simulink model "CO_laborator_04"  (R2023b)
settings: Solver=VariableStepAuto  StartTime=0.0  StopTime=100  RelTol=1e-3
values from neighbouring files (symbols this model uses):
  A = [-0.313, 56.7 0; -0.0139 -0.426 0; 0 56.7 0]    [CO_laborator_04.m]
  B = [0.232; 0.0203; 0]    [CO_laborator_04.m]
  C = [0 0 1]    [CO_laborator_04.m]
  K = lqr(A,B,Q,R)    [CO_laborator_04.m]
  Kx = K(1:3)    [CO_laborator_04.m]
  Kz = K(4)    [CO_laborator_04.m]
  N = length(t)    [CO_laborator_04.m]
settings Model: Creator=ovidiuceoca  LastModifiedBy=ovidiuceoca

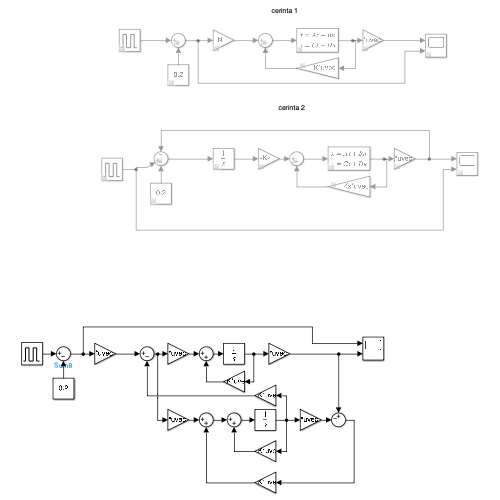
[thumbnail: Simulink's stored preview of the top-level diagram]
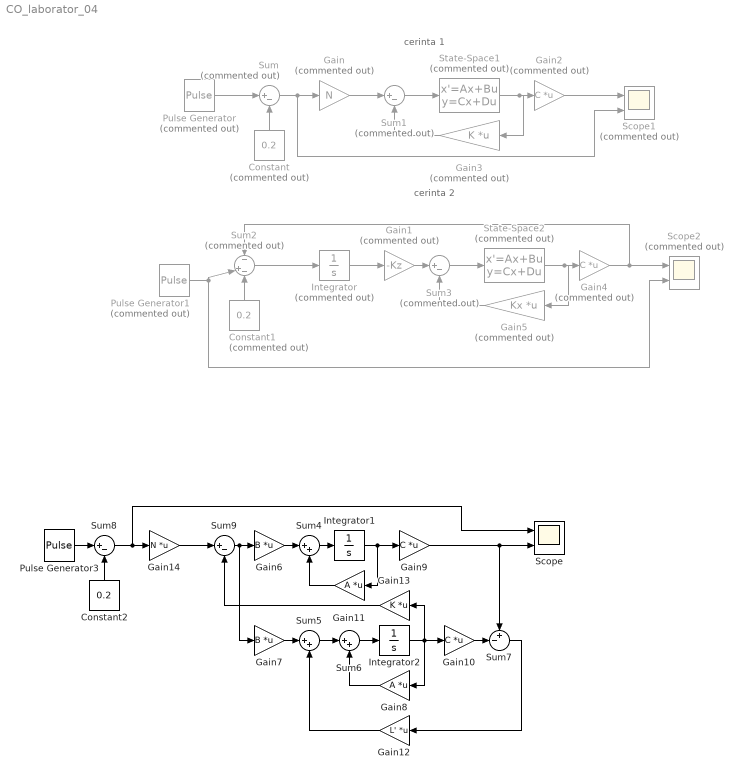
== system CO_laborator_04 ==
  note: cerinta 2
  note: cerinta 1
  Constant : Constant  Commented=on  Value=0.2
  Constant1 : Constant  Commented=on  Value=0.2
  Constant2 : Constant  Value=0.2
  Gain : Gain  Commented=on  Gain=N
  Gain1 : Gain  Commented=on  Gain=-Kz
  Gain10 : Gain  Gain=C  Multiplication=Matrix(K*u) (u vector)
  Gain11 : Gain  Gain=A  Multiplication=Matrix(K*u) (u vector)
  Gain12 : Gain  Gain=L'  Multiplication=Matrix(K*u) (u vector)
  Gain13 : Gain  Gain=K  Multiplication=Matrix(K*u) (u vector)
  Gain14 : Gain  Gain=N  Multiplication=Matrix(K*u) (u vector)
  Gain2 : Gain  Commented=on  Gain=C  Multiplication=Matrix(K*u) (u vector)
  Gain3 : Gain  Commented=on  Gain=K  Multiplication=Matrix(K*u) (u vector)
  Gain4 : Gain  Commented=on  Gain=C  Multiplication=Matrix(K*u) (u vector)
  Gain5 : Gain  Commented=on  Gain=Kx  Multiplication=Matrix(K*u) (u vector)
  Gain6 : Gain  Gain=B  Multiplication=Matrix(K*u) (u vector)
  Gain7 : Gain  Gain=B  Multiplication=Matrix(K*u) (u vector)
  Gain8 : Gain  Gain=A  Multiplication=Matrix(K*u) (u vector)
  Gain9 : Gain  Gain=C  Multiplication=Matrix(K*u) (u vector)
  Integrator : Integrator  Commented=on
  Integrator1 : Integrator
  Integrator2 : Integrator  InitialCondition=[1,2,3]
  Pulse Generator : DiscretePulseGenerator  Commented=on  PulseType=Time based  Amplitude=0.4  Period=30  PulseWidth=50  PhaseDelay=15
  Pulse Generator1 : DiscretePulseGenerator  Commented=on  PulseType=Time based  Amplitude=0.4  Period=30  PulseWidth=50  PhaseDelay=15
  Pulse Generator3 : DiscretePulseGenerator  PulseType=Time based  Amplitude=0.4  Period=30  PulseWidth=50  PhaseDelay=15
  Scope : Scope  NumInputPorts=2
  Scope1 : Scope  Commented=on  NumInputPorts=2
  Scope2 : Scope  Commented=on  NumInputPorts=2
  State-Space1 : StateSpace  Commented=on  A=A  B=B  C=eye(3)  D=[0;0;0]  InitialCondition=[1;2;3]
  State-Space2 : StateSpace  Commented=on  A=A  B=B  C=eye(3)  D=[0;0;0]  InitialCondition=0
  Sum : Sum  Commented=on  Inputs=|+-
  Sum1 : Sum  Commented=on  Inputs=|+-
  Sum2 : Sum  Commented=on  Inputs=-|+-
  Sum3 : Sum  Commented=on  Inputs=|+-
  Sum4 : Sum  Inputs=|++
  Sum5 : Sum  Inputs=|++
  Sum6 : Sum  Inputs=|++
  Sum7 : Sum  Inputs=+-|
  Sum8 : Sum  Inputs=|+-
  Sum9 : Sum  Inputs=|+-
  wires:
  Sum1/1 -> State-Space1/1
  State-Space1/1 -> Gain3/1, Gain2/1
  Gain3/1 -> Sum1/2
  Gain/1 -> Sum1/1
  Gain2/1 -> Scope1/1
  Pulse Generator/1 -> Sum/1
  Sum/1 -> Scope1/2, Gain/1
  Constant/1 -> Sum/2
  Sum2/1 -> Integrator/1
  Gain4/1 -> Sum2/1, Scope2/1
  Constant1/1 -> Sum2/3
  Pulse Generator1/1 -> Sum2/2, Scope2/2
  State-Space2/1 -> Gain5/1, Gain4/1
  Sum3/1 -> State-Space2/1
  Gain5/1 -> Sum3/2
  Gain1/1 -> Sum3/1
  Integrator/1 -> Gain1/1
  Gain6/1 -> Sum4/1
  Sum4/1 -> Integrator1/1
  Integrator1/1 -> Gain11/1, Gain9/1
  Gain11/1 -> Sum4/2
  Gain7/1 -> Sum5/1
  Sum5/1 -> Sum6/1
  Sum6/1 -> Integrator2/1
  Integrator2/1 -> Gain13/1, Gain8/1, Gain10/1
  Gain8/1 -> Sum6/2
  Gain10/1 -> Sum7/2
  Sum7/1 -> Gain12/1
  Gain12/1 -> Sum5/2
  Gain9/1 -> Sum7/1, Scope/2
  Pulse Generator3/1 -> Sum8/1
  Constant2/1 -> Sum8/2
  Gain13/1 -> Sum9/2
  Sum8/1 -> Scope/1, Gain14/1
  Sum9/1 -> Gain7/1, Gain6/1
  Gain14/1 -> Sum9/1
